simulink model "drone_failure_v2"  (R2021a)
settings: Solver=ode15s  StartTime=0.0  StopTime=35  FixedStep=0.1  RelTol=1e-3  EnableMultiTasking=on
settings Model: Creator=glembrez  LastModifiedBy=gabin
settings SolverCC: AlgebraicLoopSolver=TrustRegion  AutoInsertRateTranBlk=on
settings DataIOCC: LimitDataPoints=on
settings OptimizationCC: LifeSpan=inf
settings DebuggingCC: AllowSymbolicDim=off  SFUnexpectedBacktrackingDiag=warning  SFNoUnconditionalDefaultTransitionDiag=warning  SFExecutionAtInitializationDiag=none  ArithmeticOperatorsInVariantConditions=warning
settings SFSimCC: SimUseLocalCustomCode=off  CustomCodeUndefinedFunction=UseInterfaceOnly
settings RTWCC: RTWUseLocalCustomCode=off
settings CodeAppCC: StateflowObjectComments=on
settings GRTTargetCC: TargetLangStandard=C89/C90 (ANSI)
settings ConfigComp: CovMetricSettings=dw  CovSaveCumulativeToWorkspaceVar=on  CovSaveSingleToWorkspaceVar=on  CovExternalEMLEnable=off  CovSFcnEnable=off

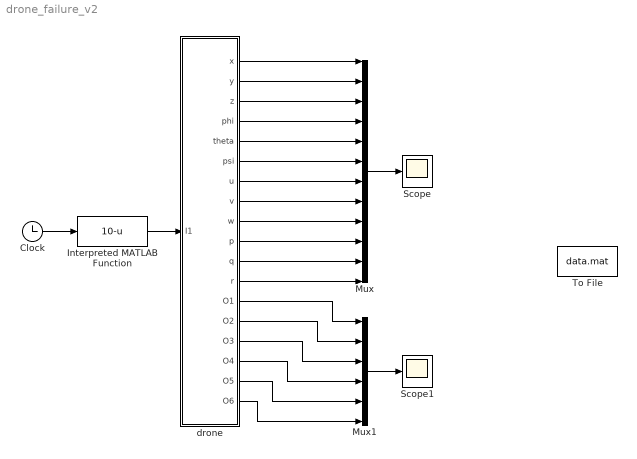
== system drone_failure_v2 ==
  Clock : Clock
  Interpreted MATLAB Function : MATLABFcn  MATLABFcn=10-u
  Mux : Mux  Inputs=12
  Mux1 : Mux  Inputs=6
  Scope : Scope
  Scope1 : Scope
  To File : ToFile  Filename=data.mat  MatrixName=X  SaveFormat=Timeseries
  drone : Stateflow chart  TreatAsAtomicUnit=on
  wires:
  drone/1(x) -> Mux/1
  Mux/1 -> Scope/1
  drone/2(y) -> Mux/2
  drone/3(z) -> Mux/3
  drone/4(phi) -> Mux/4
  drone/5(theta) -> Mux/5
  drone/6(psi) -> Mux/6
  drone/7(u) -> Mux/7
  drone/8(v) -> Mux/8
  drone/9(w) -> Mux/9
  drone/10(p) -> Mux/10
  drone/11(q) -> Mux/11
  drone/12(r) -> Mux/12
  drone/13(O1) -> Mux1/1
  drone/14(O2) -> Mux1/2
  drone/15(O3) -> Mux1/3
  drone/16(O4) -> Mux1/4
  drone/17(O5) -> Mux1/5
  drone/18(O6) -> Mux1/6
  Mux1/1 -> Scope1/1
  Clock/1 -> Interpreted MATLAB Function/1
  Interpreted MATLAB Function/1 -> drone/1(I1)

== stateflow chart drone_failure_v2/drone ==
  settings: updateMethod=CONTINUOUS
  state Drone
    state Normal_flight [parallel]
      %drone dynamic
      during:
      x_dot = cos(theta)*cos(psi)*u + (cos(psi)*sin(phi)*sin(theta)-cos(psi)*cos(phi))*v + (sin(phi)*sin(psi)+cos(phi)*cos(psi)*sin(theta))*w ;
      y_dot = cos(theta)*sin(psi)*u + (cos(theta)*cos(psi)+sin(phi)*sin(theta)*sin(psi))*v + (cos(phi)*sin(theta)*sin(psi)-sin(phi)*cos(psi))*w ;
      z_dot = -sin(theta)*u + cos(theta)*sin(phi)*v + cos(theta)*cos(phi)*w ;
      phi_dot = p+sin(phi)*tan(theta)*q+cos(phi)*tan(theta)*r ;
      theta_dot = cos(phi)*q - sin(phi)*r ;
      psi_dot = q*sin(phi)/cos(theta) + r*cos(phi)/cos(theta) ;
      u_dot = v*r-q*w-g*sin(theta)-u*(Kt+Kd*sqrt(u^2+v^2+w^2))/m ;
      v_dot = p*w-r*u+g*sin(phi)*cos(theta)-v*(Kt+Kd*sqrt(u^2+v^2+w^2))/m ;
      w_dot =q*u-p*v+g*cos(phi)*cos(theta)-w*Kd*sqrt(u^2+v^2+w^2)/m-(b*(O1^4+O2^4+O3^4+O4^4+O5^4+O6^4))/m;
      p_dot = q*r*(Iyy-Izz)/Ixx +((b*l/2 * (2*O2^4-2*O5^4+O1^4+O3^4-O4^4-O6^4))...
      -Jr*q*(-O1^2+O2^2-O3^2+O4^2-O5^2+O6^2))/Ixx;
      q_dot = p*r*(Izz-Ixx)/Iyy+((sqrt(3)*b*l/2 * (O1^4+O6^4-O3^4-O4^4))...
      +Jr*p*(-O1^2+O2^2-O3^2+O4^2-O5^2+O6^2))/Iyy ;
      r_dot = p*q*(Ixx-Iyy)/Izz+ (d*(O1^4-O2^4+O3^4-O4^4+O5^4-O6^4)...
      -Jr*2*(-O1*(O1c - O1)/0.01+O2*(O2c - O2)/0.01-O3*(O3c - O3)/0.01...
      +O4*(O4c - O4)/0.01-O5*(O5c - O5)/0.01+O6*(O6c - O6)/0.01))/Izz ;
      settings: executionOrder=1
    state Failure_detection [parallel]
      settings: executionOrder=2
      state P_correction
        during:
        O1_dot = (O1c - O1)/0.01 ;
        O2_dot = (O2c - O2)/0.01 ;
        O3_dot = (O3c - O3)/0.01 ;
        O4_dot = (O4c - O4)/0.01 ;
        O5_dot = (O5c - O5)/0.01 ;
        O6_dot = (O6c - O6)/0.01 ;
      state motor1_fails
      state sleep
      motor1_fails -> P_correction : {O1c=0;
          | O2c = (m*g/(4*b))^(1/4);
          | O3c = (m*g/(4*b))^(1/4);
          | O4c = 0;
          | O5c = (m*g/(4*b))^(1/4);
          | O6c = (m*g/(4*b))^(1/4)}
      (default) -> sleep
      sleep -> motor1_fails : [I1<0]
  data: Ixx local =5.126e-3; Iyy local =5.126e-3; Izz local =1.3e-2; l local =0.5; d local =1.140e-7; g local =9.81; m local =2.4; Kd local =7.5e-3; Kt local =3.13e-5; b local =2.98e-5; x output =0; y output =0; z output =10; phi output =0; theta output =0; psi output =0; u output =0; v output =0; w output =0; p output =0; q output =0; r output =0; Jr local =4.2e-6; M_phi local =0; M_theta local =0; M_psi local =0; O_R local =0; O_R_d local =0; O1c local =19.05; O2c local =19.05; O3c local =19.05; O4c local =19.05; O5c local =19.05; O6c local =19.05; O1 output =19.05; O2 output =19.05; O3 output =19.05; O4 output =19.05; O5 output =19.05; O6 output =19.05; Tt local =23.544; I1 input
  data x settings: updateMethod=SF_CONTINUOUS_TIME_DATA
  data y settings: updateMethod=SF_CONTINUOUS_TIME_DATA
  data z settings: updateMethod=SF_CONTINUOUS_TIME_DATA
  data phi settings: updateMethod=SF_CONTINUOUS_TIME_DATA
  data theta settings: updateMethod=SF_CONTINUOUS_TIME_DATA
  data psi settings: updateMethod=SF_CONTINUOUS_TIME_DATA
  data u settings: updateMethod=SF_CONTINUOUS_TIME_DATA
  data v settings: updateMethod=SF_CONTINUOUS_TIME_DATA
  data w settings: updateMethod=SF_CONTINUOUS_TIME_DATA
  data p settings: updateMethod=SF_CONTINUOUS_TIME_DATA
  data q settings: updateMethod=SF_CONTINUOUS_TIME_DATA
  data r settings: updateMethod=SF_CONTINUOUS_TIME_DATA
  data O1 settings: updateMethod=SF_CONTINUOUS_TIME_DATA
  data O2 settings: updateMethod=SF_CONTINUOUS_TIME_DATA
  data O3 settings: updateMethod=SF_CONTINUOUS_TIME_DATA
  data O4 settings: updateMethod=SF_CONTINUOUS_TIME_DATA
  data O5 settings: updateMethod=SF_CONTINUOUS_TIME_DATA
  data O6 settings: updateMethod=SF_CONTINUOUS_TIME_DATA
